simulink model "plant"  (R2015b)
settings: Solver=FixedStepAuto  StartTime=0.0  StopTime=10  FixedStep=0.001  RelTol=1e-3
values from neighbouring files (symbols this model uses):
  butterworthOrder = 1    [prerunScript.m]
  FP_c = x(1,1)    [checkPFvsL.m]    (also in passForceParams.m = 0.000395332869306)
  FP_k = x(1,2)    [checkPFvsL.m]    (also in passForceParams.m = 0.132380005179)
  FP_lr = x(1,3)    [checkPFvsL.m]    (also in passForceParams.m = -0.491551555037)
  lambda0 = [[0.00350486];[0.06666161];[0.14223155];[0.17875788];[0.09072633];[0.19503137];[0.07421535];[0.06014449];[0.07737726];[0.15431079];[0.05739210];[0.08251990];[0.05507007];[0.05698303];[0.06408346];[0.06303047];[0.05043992];[0.06209895];[0.05972867];[0.06428054];[0.05550584];[0.06070605];[0.04113306];[0.06599153];[0.06665474];[0.06653758];[0.07028198];[0.07750712];[0.04229977];[0.06486173];[0.064262 ...(+251 chars)    [prerunScript.m]
  ldotECoeffs = ldotCoeffs.ldotE    [prerunScript.m]
  ldotSCoeffs = ldotCoeffs.ldotS    [prerunScript.m]
  optimalLambda = [[0.027];[0.0713];[0.1157];[0.1321];[0.0858];[0.1726];      [0.0932];[0.0976];[0.1078];[0.1367];[0.0585];[0.081];[0.0622];[0.07];      [0.065];[0.0724];[0.0626];[0.0675];[0.0589];[0.0675];[0.054];[0.0628];      [0.0509];[0.0749];[0.0749];[0.0835];[0.0798];[0.0835];[0.0515];[0.0749];      [0.0736];[0.0552];[0.0755];[0.254];[0.2324];[0.2789];[0.1442];[0.1385];      [0.1385];[0.0638];[0.0282];[0.0492 ...(+78 chars)    [checkPFvsL.m]    (also in prerunScript.m)
  rhoECoeffs = zeros(50,degree+1)    [fit_moments.m]    (also in prerunScript.m = rhoCoeffs.rhoECoeffs; rhoCoeffs.mat = [1.24545301291e-20 0 -1.29464465569e-20 -1.29464465569e-20 -)
  rhoSCoeffs = zeros(50,degree+1)    [fit_moments.m]    (also in prerunScript.m = rhoCoeffs.rhoSCoeffs; rhoCoeffs.mat = [0 0 -4.82961585868e-21 1.75624779335e-24 0 0 1.43054523333e)
  uANC_p_a = 0    [setPCurla.m]    (also in setPRest.m; setPRestSLock.m; setPSweep.m)
  uANC_p_d = 1    [setPCurla.m]    (also in setPRest.m; setPRestSLock.m; setPSweep.m)
  uANC_p_p = 10    [setPCurla.m]    (also in setPRest.m; setPRestSLock.m; setPSweep.m)
  uANC_p_w = 20    [setPCurla.m]    (also in setPRest.m; setPRestSLock.m; setPSweep.m)
  uBRD_a = 25    [setPCurla.m]    (also in setPRest.m = 0; setPRestSLock.m = 0; setPSweep.m = 5; setPTPEC2.m = 0)
  uBRD_b = 0    [setPCurla.m]    (also in setPRest.m; setPRestSLock.m; setPSweep.m; setPTPEC2.m)
  uBRD_f = pi/10*3    (= 0.942477796077)    [setPCurla.m]    (also in setPRest.m; setPRestSLock.m; setPSweep.m; setPTPEC2.m)
  uBRD_p = 0    [setPCurla.m]    (also in setPRest.m; setPRestSLock.m; setPSweep.m; setPTPEC2.m)
  uTRIlong_a = 1140    [setPCurla.m]    (also in setPRest.m = 0; setPRestSLock.m = 0; setPSweep.m = 0; setPTPEC2.m = 0)
  uTRIlong_b = 0    [setPCurla.m]    (also in setPRest.m; setPRestSLock.m; setPSweep.m; setPTPEC2.m)
  uTRIlong_f = pi/10*3    (= 0.942477796077)    [setPCurla.m]    (also in setPRest.m; setPRestSLock.m; setPSweep.m; setPTPEC2.m)
  uTRIlong_p = pi    (= 3.14159265359)    [setPCurla.m]    (also in setPRest.m; setPRestSLock.m; setPSweep.m; setPTPEC2.m)
libraries: dsparch4 x50
settings Model: Creator=awni1  LastModifiedBy=hawni
settings DataIOCC: LimitDataPoints=off  SaveFormat=Array
settings HardwareCC: ProdBitPerPointer=32  ProdLargestAtomicFloat=None  ProdIntDivRoundTo=Undefined  ProdEndianess=Unspecified  ProdWordSize=32  ProdHWDeviceType=32-bit Generic
settings GRTTargetCC: GeneratePreprocessorConditionals=Disable all
settings ConfigComp: CovModelRefEnable=Off

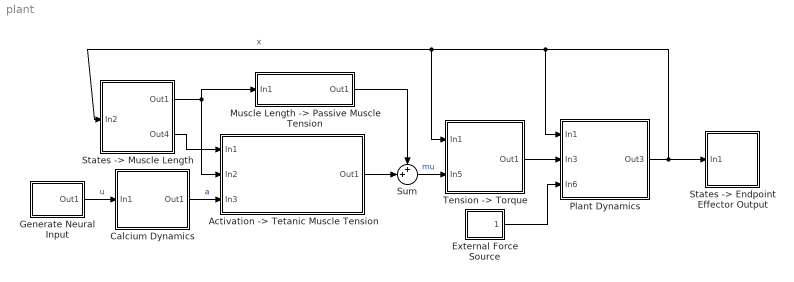
== system plant ==
  "Activation -> Tetanic Muscle Tension" : Subsystem
  Calcium Dynamics : Subsystem
  External Force Source : Subsystem
  Generate Neural Input : Subsystem
  "Muscle Length -> Passive Muscle Tension" : Subsystem
  Plant Dynamics : Subsystem
  "States -> Endpoint Effector Output" : Subsystem
  "States -> Muscle Length" : Subsystem
  Sum : Sum  Inputs=++|
  "Tension -> Torque" : Subsystem
  wires:
  Plant Dynamics/1(Out3) -> "States -> Muscle Length"/1(In2), "Tension -> Torque"/1(In1), Plant Dynamics/1(In1), "States -> Endpoint Effector Output"/1(In1)  "x"
  Calcium Dynamics/1(Out1) -> "Activation -> Tetanic Muscle Tension"/3(In3)  "a"
  "Activation -> Tetanic Muscle Tension"/1(Out1) -> Sum/2
  "States -> Muscle Length"/1(Out1) -> "Muscle Length -> Passive Muscle Tension"/1(In1), "Activation -> Tetanic Muscle Tension"/2(In2)
  "States -> Muscle Length"/2(Out4) -> "Activation -> Tetanic Muscle Tension"/1(In1)
  "Muscle Length -> Passive Muscle Tension"/1(Out1) -> Sum/1
  Sum/1 -> "Tension -> Torque"/2(In5)  "mu"
  "Tension -> Torque"/1(Out1) -> Plant Dynamics/2(In3)
  External Force Source/1(Out1) -> Plant Dynamics/3(In6)
  Generate Neural Input/1(Out1) -> Calcium Dynamics/1(In1)  "u"

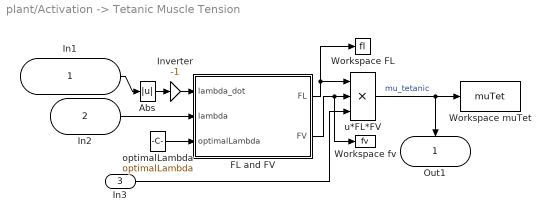
== system plant/Activation -> Tetanic Muscle Tension ==
  In1 : Inport
  In2 : Inport  Port=2
  In3 : Inport  Port=3
  Abs : Abs
  FL and FV : MATLAB Function  TreatAsAtomicUnit=on
  Inverter : Gain  Gain=-1
  Workspace FL : ToWorkspace  VariableName=fl  SampleTime=-1
  Workspace fv : ToWorkspace  VariableName=fv  SampleTime=-1
  Workspace muTet : ToWorkspace  VariableName=muTet  SampleTime=-1
  optimalLambda : Constant  Value=optimalLambda
  u*FL*FV : Product  Inputs=3
  Out1 : Outport
  wires:
  In2/1 -> FL and FV/2(lambda)
  In3/1 -> u*FL*FV/3
  In1/1 -> Abs/1
  FL and FV/1(FL) -> Workspace FL/1, u*FL*FV/1
  FL and FV/2(FV) -> Workspace fv/1, u*FL*FV/2
  optimalLambda/1 -> FL and FV/3(optimalLambda)
  Abs/1 -> Inverter/1
  Inverter/1 -> FL and FV/1(lambda_dot)
  u*FL*FV/1 -> Workspace muTet/1, Out1/1  "mu_tetanic"

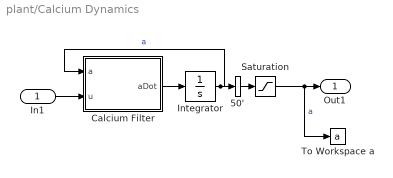
== system plant/Calcium Dynamics ==
  In1 : Inport
  50' : SignalSpecification  Dimensions=50
  Calcium Filter : MATLAB Function  TreatAsAtomicUnit=on
  Integrator : Integrator
  Saturation : Saturate  UpperLimit=inf  LowerLimit=0
  To Workspace a : ToWorkspace  VariableName=a  SampleTime=-1
  Out1 : Outport
  wires:
  In1/1 -> Calcium Filter/2(u)
  Saturation/1 -> To Workspace a/1, Out1/1  "a"
  50'/1 -> Saturation/1
  Calcium Filter/1(aDot) -> Integrator/1
  Integrator/1 -> Calcium Filter/1(a), 50'/1  "a"

== system plant/External Force Source ==
  Mux1 : Mux  Inputs=2
  Out1 : Outport
  wires:
  Mux1/1 -> Out1/1  "fE"

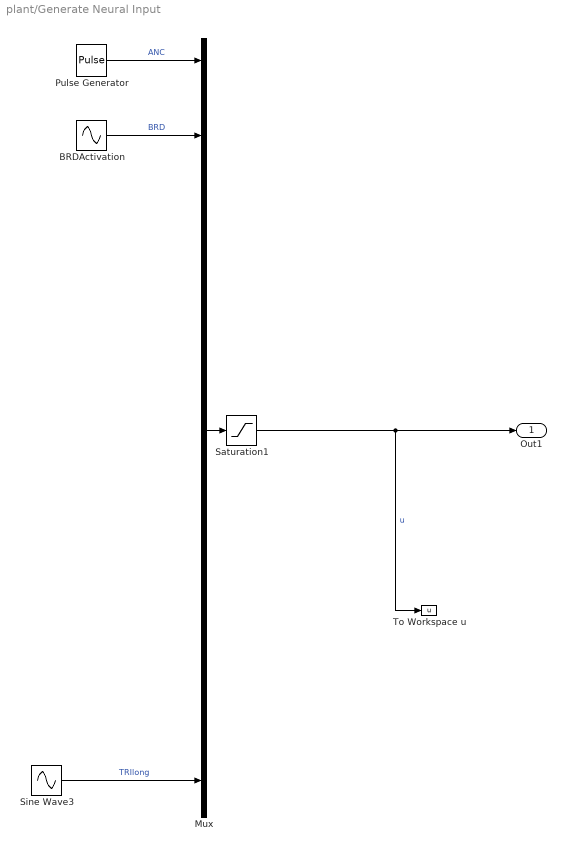
== system plant/Generate Neural Input ==
  BRDActivation : Sin  Amplitude=uBRD_a  Bias=uBRD_b  Frequency=uBRD_f  Phase=uBRD_p  SampleTime=0
  Mux : Mux  Inputs=50
  Pulse Generator : DiscretePulseGenerator  PulseType=Time based  Amplitude=uANC_p_a  Period=uANC_p_p  PulseWidth=uANC_p_w  PhaseDelay=uANC_p_d
  Saturation1 : Saturate  UpperLimit=1  LowerLimit=0
  Sine Wave3 : Sin  Amplitude=uTRIlong_a  Bias=uTRIlong_b  Frequency=uTRIlong_f  Phase=uTRIlong_p  SampleTime=0
  To Workspace u : ToWorkspace  VariableName=u  SampleTime=-1
  Out1 : Outport
  wires:
  ? -> Mux/41
  ? -> Mux/11
  ? -> Mux/23
  ? -> Mux/27
  ? -> Mux/3
  ? -> Mux/8
  ? -> Mux/29
  ? -> Mux/18
  ? -> Mux/19
  ? -> Mux/28
  ? -> Mux/26
  ? -> Mux/43
  ? -> Mux/33
  ? -> Mux/32
  ? -> Mux/17
  ? -> Mux/37
  ? -> Mux/42
  ? -> Mux/47
  ? -> Mux/48
  ? -> Mux/9
  ? -> Mux/16
  ? -> Mux/13
  ? -> Mux/4
  ? -> Mux/46
  ? -> Mux/22
  ? -> Mux/39
  ? -> Mux/7
  ? -> Mux/21
  ? -> Mux/24
  ? -> Mux/34
  ? -> Mux/44
  ? -> Mux/5
  ? -> Mux/15
  ? -> Mux/25
  ? -> Mux/35
  ? -> Mux/45
  ? -> Mux/38  "PEC2"
  Sine Wave3/1 -> Mux/49  "TRIlong"
  Pulse Generator/1 -> Mux/1  "ANC"
  Mux/1 -> Saturation1/1
  Saturation1/1 -> Out1/1, To Workspace u/1  "u"
  ? -> Mux/36
  ? -> Mux/2
  ? -> Mux/12
  ? -> Mux/31
  ? -> Mux/14
  BRDActivation/1 -> Mux/6  "BRD"

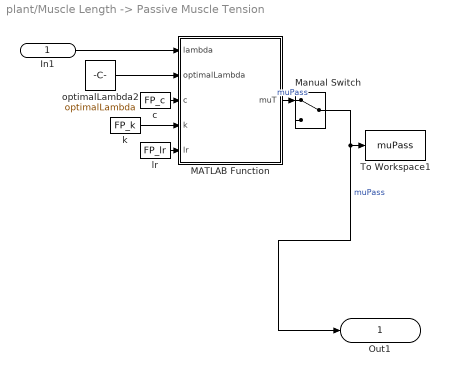
== system plant/Muscle Length -> Passive Muscle Tension ==
  In1 : Inport
  MATLAB Function : MATLAB Function  TreatAsAtomicUnit=on
  Manual Switch : ManualSwitch
  To Workspace1 : ToWorkspace  VariableName=muPass  SampleTime=-1
  c : Constant  Value=FP_c
  k : Constant  Value=FP_k
  lr : Constant  Value=FP_lr
  optimalLambda2 : Constant  Value=optimalLambda
  Out1 : Outport
  wires:
  In1/1 -> MATLAB Function/1(lambda)
  c/1 -> MATLAB Function/3(c)
  k/1 -> MATLAB Function/4(k)
  lr/1 -> MATLAB Function/5(lr)
  optimalLambda2/1 -> MATLAB Function/2(optimalLambda)
  MATLAB Function/1(muT) -> Manual Switch/1  "muPass"
  Manual Switch/1 -> Out1/1, To Workspace1/1  "muPass"

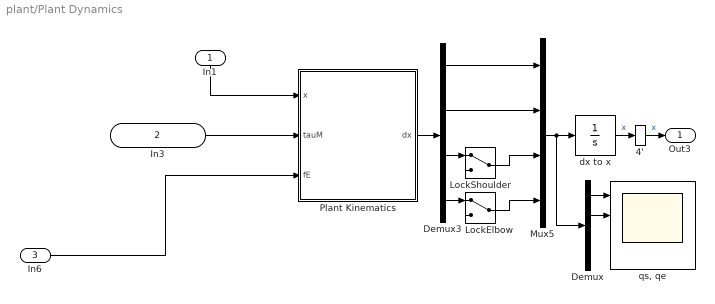
== system plant/Plant Dynamics ==
  In1 : Inport
  In3 : Inport  Port=2
  In6 : Inport  Port=3
  4' : SignalSpecification  Dimensions=4
  Demux : Demux
  Demux3 : Demux
  LockElbow : ManualSwitch
  LockShoulder : ManualSwitch
  Mux5 : Mux
  Plant Kinematics : MATLAB Function  TreatAsAtomicUnit=on
  dx to x : Integrator  InitialCondition=[90,0,0,0]
  "qs, qe" : Scope  NumInputPorts=4
  Out3 : Outport
  wires:
  In3/1 -> Plant Kinematics/2(tauM)
  In1/1 -> Plant Kinematics/1(x)
  In6/1 -> Plant Kinematics/3(fE)
  Plant Kinematics/1(dx) -> Demux3/1
  Demux3/4 -> LockElbow/1
  LockShoulder/1 -> Mux5/3
  Demux3/3 -> LockShoulder/1
  LockElbow/1 -> Mux5/4
  Demux3/1 -> Mux5/1
  Demux3/2 -> Mux5/2
  Demux/2 -> "qs, qe"/2
  Mux5/1 -> Demux/1, dx to x/1
  dx to x/1 -> 4'/1  "x"
  4'/1 -> Out3/1  "x"
  Demux/1 -> "qs, qe"/1

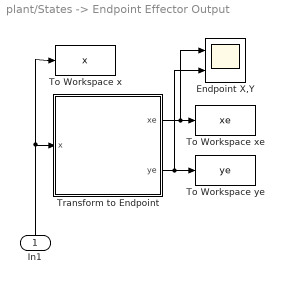
== system plant/States -> Endpoint Effector Output ==
  In1 : Inport
  Endpoint X,Y : Scope  NumInputPorts=2
  To Workspace x : ToWorkspace  VariableName=x  SampleTime=-1
  To Workspace xe : ToWorkspace  VariableName=xe  SampleTime=-1
  To Workspace ye : ToWorkspace  VariableName=ye  SampleTime=-1
  Transform to Endpoint : MATLAB Function  TreatAsAtomicUnit=on
  wires:
  In1/1 -> To Workspace x/1, Transform to Endpoint/1(x)
  Transform to Endpoint/1(xe) -> Endpoint X,Y/1, To Workspace xe/1
  Transform to Endpoint/2(ye) -> Endpoint X,Y/2, To Workspace ye/1

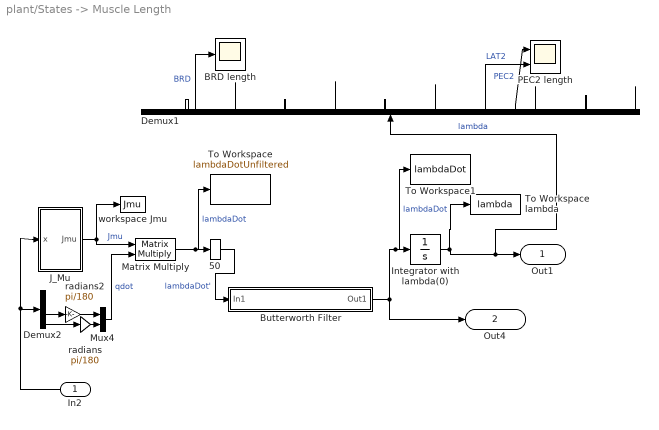
== system plant/States -> Muscle Length ==
  In2 : Inport
  50 : SignalSpecification  Dimensions=50
  BRD length : Scope
  Butterworth Filter : Subsystem
  Demux1 : Demux  Outputs=50
  Demux2 : Demux
  Integrator with lambda(0) : Integrator  InitialCondition=lambda0
  J_Mu : Subsystem
  Matrix Multiply : Product  Multiplication=Matrix(*)
  Mux4 : Mux  Inputs=2
  PEC2 length : Scope  NumInputPorts=2
  To Workspace : ToWorkspace  VariableName=lambdaDotUnfiltered  SampleTime=-1
  To Workspace lambda : ToWorkspace  VariableName=lambda  SampleTime=-1
  To Workspace1 : ToWorkspace  VariableName=lambdaDot  SampleTime=-1
  radians : Gain  Gain=pi/180
  radians2 : Gain  Gain=pi/180
  workspace Jmu : ToWorkspace  VariableName=Jmu  SampleTime=-1
  Out1 : Outport
  Out4 : Outport  Port=2
  wires:
  In2/1 -> Demux2/1, J_Mu/1(x)
  J_Mu/1(Jmu) -> workspace Jmu/1, Matrix Multiply/1  "Jmu"
  Mux4/1 -> Matrix Multiply/2  "qdot"
  Matrix Multiply/1 -> To Workspace/1, 50/1  "lambdaDot"
  Integrator with lambda(0)/1 -> To Workspace lambda/1, Demux1/1, Out1/1  "lambda"
  Demux2/3 -> radians2/1
  radians/1 -> Mux4/2
  radians2/1 -> Mux4/1
  Demux2/4 -> radians/1
  Demux1/6 -> BRD length/1  "BRD"
  Demux1/5 -> ?
  Demux1/10 -> ?
  Demux1/15 -> ?
  Demux1/20 -> ?
  Demux1/25 -> ?
  Demux1/30 -> ?
  Demux1/40 -> ?
  Demux1/45 -> ?
  Demux1/50 -> ?
  Demux1/38 -> PEC2 length/1  "PEC2"
  Demux1/35 -> PEC2 length/2  "LAT2"
  50/1 -> Butterworth Filter/1(In1)  "lambdaDot'"
  Butterworth Filter/1(Out1) -> Out4/1, To Workspace1/1, Integrator with lambda(0)/1  "lambdaDot"

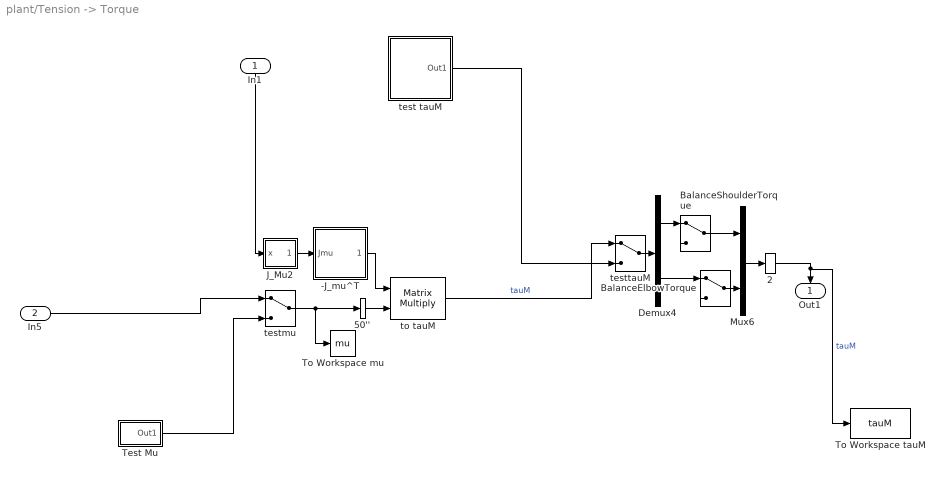
== system plant/Tension -> Torque ==
  In1 : Inport
  In5 : Inport  Port=2
  -J_mu^T : MATLAB Function  TreatAsAtomicUnit=on
  2 : SignalSpecification  Dimensions=2
  50'' : SignalSpecification  Dimensions=50
  BalanceElbowTorque : ManualSwitch
  BalanceShoulderTorque : ManualSwitch
  Demux4 : Demux  Outputs=2
  J_Mu2 : Subsystem
  Mux6 : Mux  Inputs=2
  Test Mu : Subsystem
  To Workspace mu : ToWorkspace  VariableName=mu  SampleTime=-1
  To Workspace tauM : ToWorkspace  VariableName=tauM  SampleTime=-1
  test tauM : Subsystem
  testmu : ManualSwitch
  testtauM : ManualSwitch
  to tauM : Product  Multiplication=Matrix(*)
  Out1 : Outport
  wires:
  In5/1 -> testmu/1
  In1/1 -> J_Mu2/1(x)
  2/1 -> To Workspace tauM/1, Out1/1  "tauM"
  testmu/1 -> 50''/1, To Workspace mu/1
  -J_mu^T/1(JmuT) -> to tauM/1
  J_Mu2/1(Jmu) -> -J_mu^T/1(Jmu)
  to tauM/1 -> testtauM/1  "tauM"
  50''/1 -> to tauM/2
  Mux6/1 -> 2/1
  testtauM/1 -> Demux4/1
  BalanceShoulderTorque/1 -> Mux6/1
  BalanceElbowTorque/1 -> Mux6/2
  Demux4/1 -> BalanceShoulderTorque/1
  Demux4/2 -> BalanceElbowTorque/1
  Test Mu/1(Out1) -> testmu/2
  test tauM/1(Out1) -> testtauM/2

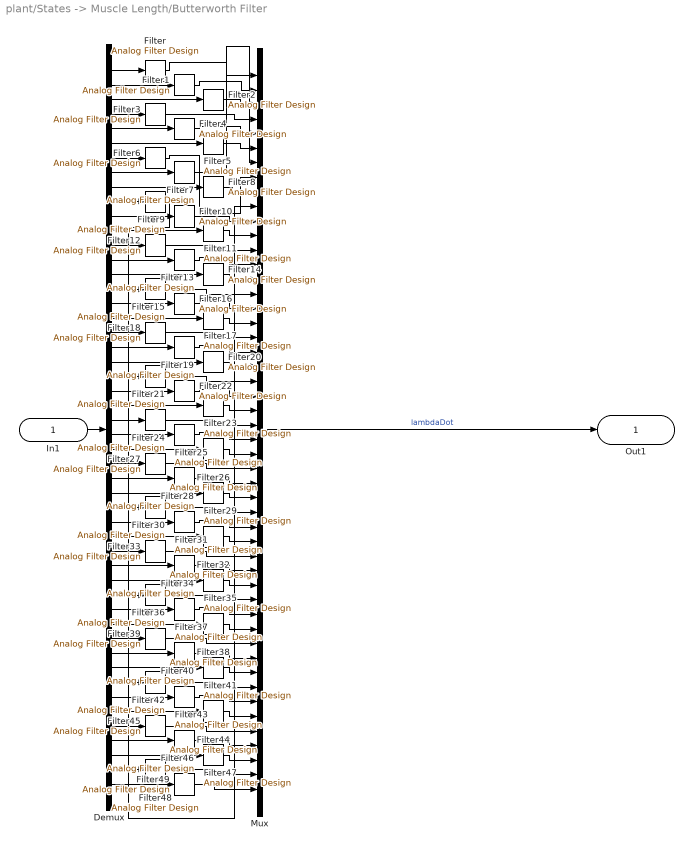
== system plant/States -> Muscle Length/Butterworth Filter ==
  In1 : Inport
  Demux : Demux  Outputs=50
  Filter{,1..49} (50 alike) : dsparch4/Analog Filter Design  method=Butterworth  filttype=Lowpass  N=butterworthOrder  Wlo=butterworthCutoffFreq  Whi=80  Rp=2  Rs=40
  Mux : Mux  Inputs=50
  Out1 : Outport
  wires:
  In1/1 -> Demux/1
  Demux/1 -> Filter/1
  Demux/2 -> Filter1/1
  Demux/3 -> Filter2/1
  Demux/4 -> Filter3/1
  Demux/5 -> Filter4/1
  Demux/6 -> Filter5/1
  Demux/9 -> Filter8/1
  Demux/8 -> Filter7/1
  Demux/7 -> Filter6/1
  Demux/10 -> Filter9/1
  Demux/11 -> Filter10/1
  Demux/12 -> Filter11/1
  Demux/13 -> Filter12/1
  Demux/14 -> Filter13/1
  Demux/15 -> Filter14/1
  Demux/16 -> Filter15/1
  Demux/17 -> Filter16/1
  Demux/18 -> Filter17/1
  Demux/19 -> Filter18/1
  Demux/20 -> Filter19/1
  Demux/21 -> Filter20/1
  Demux/22 -> Filter21/1
  Demux/23 -> Filter22/1
  Demux/24 -> Filter23/1
  Demux/26 -> Filter25/1
  Demux/25 -> Filter24/1
  Demux/27 -> Filter26/1
  Demux/28 -> Filter27/1
  Demux/29 -> Filter28/1
  Demux/30 -> Filter29/1
  Demux/31 -> Filter30/1
  Demux/32 -> Filter31/1
  Demux/33 -> Filter32/1
  Demux/34 -> Filter33/1
  Demux/35 -> Filter34/1
  Demux/36 -> Filter35/1
  Demux/37 -> Filter36/1
  Demux/38 -> Filter37/1
  Demux/39 -> Filter38/1
  Demux/40 -> Filter39/1
  Demux/41 -> Filter40/1
  Demux/42 -> Filter41/1
  Demux/43 -> Filter42/1
  Demux/44 -> Filter43/1
  Demux/45 -> Filter44/1
  Demux/47 -> Filter46/1
  Demux/46 -> Filter45/1
  Demux/48 -> Filter47/1
  Demux/49 -> Filter48/1
  Demux/50 -> Filter49/1
  Mux/1 -> Out1/1  "lambdaDot"
  Filter/1 -> Mux/1
  Filter1/1 -> Mux/2
  Filter2/1 -> Mux/3
  Filter3/1 -> Mux/4
  Filter4/1 -> Mux/5
  Filter5/1 -> Mux/6
  Filter6/1 -> Mux/7
  Filter7/1 -> Mux/8
  Filter8/1 -> Mux/9
  Filter9/1 -> Mux/10
  Filter10/1 -> Mux/11
  Filter11/1 -> Mux/12
  Filter12/1 -> Mux/13
  Filter13/1 -> Mux/14
  Filter14/1 -> Mux/15
  Filter15/1 -> Mux/16
  Filter16/1 -> Mux/17
  Filter17/1 -> Mux/18
  Filter18/1 -> Mux/19
  Filter19/1 -> Mux/20
  Filter20/1 -> Mux/21
  Filter21/1 -> Mux/22
  Filter22/1 -> Mux/23
  Filter23/1 -> Mux/24
  Filter24/1 -> Mux/25
  Filter25/1 -> Mux/26
  Filter26/1 -> Mux/27
  Filter27/1 -> Mux/28
  Filter28/1 -> Mux/29
  Filter29/1 -> Mux/30
  Filter30/1 -> Mux/31
  Filter31/1 -> Mux/32
  Filter32/1 -> Mux/33
  Filter33/1 -> Mux/34
  Filter34/1 -> Mux/35
  Filter35/1 -> Mux/36
  Filter36/1 -> Mux/37
  Filter37/1 -> Mux/38
  Filter38/1 -> Mux/39
  Filter39/1 -> Mux/40
  Filter40/1 -> Mux/41
  Filter41/1 -> Mux/42
  Filter42/1 -> Mux/43
  Filter43/1 -> Mux/44
  Filter44/1 -> Mux/45
  Filter45/1 -> Mux/46
  Filter46/1 -> Mux/47
  Filter47/1 -> Mux/48
  Filter48/1 -> Mux/49
  Filter49/1 -> Mux/50

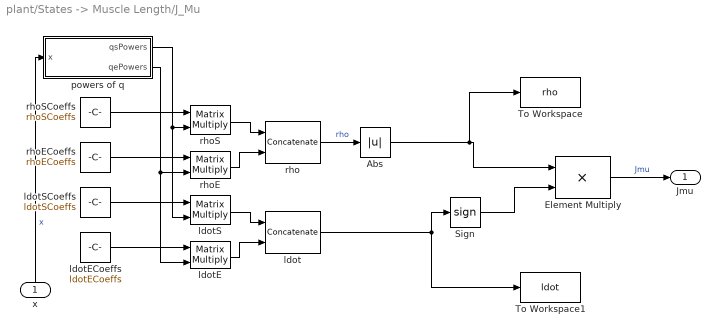
== system plant/States -> Muscle Length/J_Mu ==
  x : Inport  PortDimensions=4
  Abs : Abs
  Element Multiply : Product
  Sign : Signum
  To Workspace : ToWorkspace  VariableName=rho  SampleTime=-1
  To Workspace1 : ToWorkspace  VariableName=ldot  SampleTime=-1
  ldot : Concatenate  Mode=Multidimensional array  ConcatenateDimension=2
  ldotE : Product  Multiplication=Matrix(*)
  ldotECoeffs : Constant  Value=ldotECoeffs
  ldotS : Product  Multiplication=Matrix(*)
  ldotSCoeffs : Constant  Value=ldotSCoeffs
  powers of q : MATLAB Function  TreatAsAtomicUnit=on
  rho : Concatenate  Mode=Multidimensional array  ConcatenateDimension=2
  rhoE : Product  Multiplication=Matrix(*)
  rhoECoeffs : Constant  Value=rhoECoeffs
  rhoS : Product  Multiplication=Matrix(*)
  rhoSCoeffs : Constant  Value=rhoSCoeffs
  Jmu : Outport
  wires:
  powers of q/1(qsPowers) -> ldotS/2, rhoS/2
  rhoECoeffs/1 -> rhoE/1
  powers of q/2(qePowers) -> ldotE/2, rhoE/2
  x/1 -> powers of q/1(x)  "x"
  rhoS/1 -> rho/1
  rhoSCoeffs/1 -> rhoS/1
  rhoE/1 -> rho/2
  ldotS/1 -> ldot/1
  ldotE/1 -> ldot/2
  ldotSCoeffs/1 -> ldotS/1
  ldotECoeffs/1 -> ldotE/1
  Element Multiply/1 -> Jmu/1  "Jmu"
  ldot/1 -> Sign/1, To Workspace1/1
  rho/1 -> Abs/1  "rho"
  Abs/1 -> To Workspace/1, Element Multiply/1
  Sign/1 -> Element Multiply/2

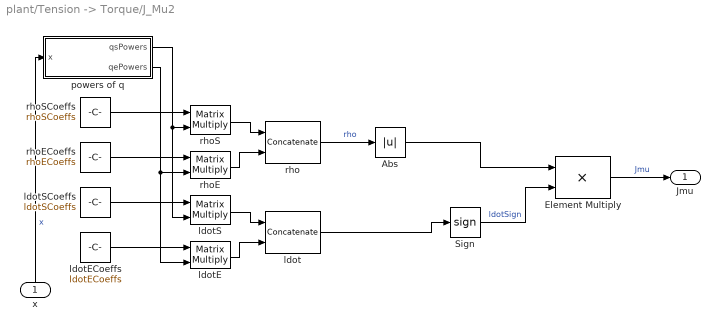
== system plant/Tension -> Torque/J_Mu2 ==
  x : Inport  PortDimensions=4
  Abs : Abs
  Element Multiply : Product
  Sign : Signum
  ldot : Concatenate  Mode=Multidimensional array  ConcatenateDimension=2
  ldotE : Product  Multiplication=Matrix(*)
  ldotECoeffs : Constant  Value=ldotECoeffs
  ldotS : Product  Multiplication=Matrix(*)
  ldotSCoeffs : Constant  Value=ldotSCoeffs
  powers of q : MATLAB Function  TreatAsAtomicUnit=on
  rho : Concatenate  Mode=Multidimensional array  ConcatenateDimension=2
  rhoE : Product  Multiplication=Matrix(*)
  rhoECoeffs : Constant  Value=rhoECoeffs
  rhoS : Product  Multiplication=Matrix(*)
  rhoSCoeffs : Constant  Value=rhoSCoeffs
  Jmu : Outport
  wires:
  powers of q/1(qsPowers) -> ldotS/2, rhoS/2
  rhoECoeffs/1 -> rhoE/1
  powers of q/2(qePowers) -> ldotE/2, rhoE/2
  x/1 -> powers of q/1(x)  "x"
  rhoS/1 -> rho/1
  rhoSCoeffs/1 -> rhoS/1
  rhoE/1 -> rho/2
  ldotS/1 -> ldot/1
  ldotE/1 -> ldot/2
  ldotSCoeffs/1 -> ldotS/1
  ldotECoeffs/1 -> ldotE/1
  Sign/1 -> Element Multiply/2  "ldotSign"
  Element Multiply/1 -> Jmu/1  "Jmu"
  ldot/1 -> Sign/1
  rho/1 -> Abs/1  "rho"
  Abs/1 -> Element Multiply/1

== system plant/Tension -> Torque/Test Mu ==
  Manual Switch : ManualSwitch  CurrentSetting=0
  Mux3 : Mux  Inputs=50
  Sine Wave1 : Sin  Frequency=2*pi/10  SampleTime=0
  Step1 : Step  Time=0  After=0  SampleTime=0
  Sum1 : Sum  Inputs=++|
  Out1 : Outport
  wires:
  ? -> Mux3/42
  Mux3/1 -> Out1/1  "testMu"
  ? -> Mux3/49
  ? -> Mux3/7
  ? -> Mux3/41
  ? -> Mux3/30
  ? -> Mux3/29
  ? -> Mux3/15
  ? -> Mux3/22
  ? -> Mux3/44
  ? -> Mux3/4
  ? -> Mux3/16
  ? -> Mux3/23
  ? -> Mux3/43
  ? -> Mux3/20
  ? -> Mux3/2
  ? -> Mux3/5
  ? -> Mux3/21
  ? -> Mux3/1
  ? -> Mux3/33
  ? -> Mux3/34
  ? -> Mux3/19
  ? -> Mux3/32
  ? -> Mux3/31
  ? -> Mux3/14
  ? -> Mux3/8
  ? -> Mux3/11
  ? -> Mux3/18
  ? -> Mux3/17
  ? -> Mux3/40
  ? -> Mux3/12
  ? -> Mux3/28
  ? -> Mux3/13
  ? -> Mux3/50
  ? -> Mux3/24
  ? -> Mux3/9
  ? -> Mux3/35
  ? -> Mux3/47
  ? -> Mux3/10
  ? -> Mux3/25
  ? -> Mux3/39
  ? -> Mux3/26
  ? -> Mux3/37
  ? -> Mux3/38
  ? -> Mux3/27
  ? -> Mux3/36
  ? -> Mux3/45
  ? -> Mux3/48
  ? -> Mux3/46
  ? -> Mux3/3
  Step1/1 -> Sum1/1
  Sine Wave1/1 -> Sum1/2
  Manual Switch/1 -> Mux3/6  "BRD"
  Sum1/1 -> Manual Switch/1

== system plant/Tension -> Torque/test tauM ==
  Mux2 : Mux  Inputs=2
  tauS : Sin  Amplitude=0.02  Frequency=2*pi/10  SampleTime=0
  Out1 : Outport
  wires:
  Mux2/1 -> Out1/1  "test_tauM"
  tauS/1 -> Mux2/2

== matlab function plant/States -> Endpoint Effector Output/Transform to Endpoint ==
  data: x input; xe output; ye output
function [xe,ye]= toEndEffectorXY(x)
% init
    Ls=0.31;
    Le=0.34;
% translate
xe = cos((x(1)*pi/180))*Ls+Le*cos((x(1)*pi/180)+(x(2)*pi/180));
ye = sin((x(1)*pi/180))*Ls+Le*sin((x(1)*pi/180)+(x(2)*pi/180));

== matlab function plant/Plant Dynamics/Plant Kinematics ==
  data: x input; dx output; tauM input; fE input
function dx = armKinematics(x, tauM, fE)
    % define constants
    is=0.0141;
    ie=0.0188;
    lms=0.165;
    lme=0.19;
    Ls=0.31;
    Le=0.34;
    ms=1.93;
    me=1.52;

    % define dx as a vector 
    dx=zeros(4,1);
    
    dx(1) = x(3);
    dx(2) = x(4);
    dx(3) = -((fE(1)*ie - fE(2)*ie + fE(1)*is + fE(1)*lme^2*me - fE(2)*lme^2 * ...
        me + fE(1)*Ls^2*me + fE(1)*lms^2*ms + ie*tauM(1) + is*tauM(1) + ... 
        lme^2*me*tauM(1) + Ls^2*me*tauM(1) + lms^2*ms*tauM(1) - ie* ...
        tauM(2) - lme^2*me*tauM(2) + fE(1)*lme*Ls*me*cos((x(2)*pi/180)) - fE(2) ...
        *lme*Ls*me*cos((x(2)*pi/180)) + lme*Ls*me*tauM(1)*cos((x(2)*pi/180)) - lme*Ls*me* ...
        tauM(2)*cos((x(2)*pi/180)) + ie*lme*Ls*me*((x(4)*pi/180))^2*sin((x(2)*pi/180)) + is*lme*Ls* ...
        me*((x(4)*pi/180))^2*sin((x(2)*pi/180)) + lme^3*Ls*me^2*((x(4)*pi/180))^2*sin((x(2)*pi/180)) + lme* ...
        Ls^3*me^2*((x(4)*pi/180))^2*sin((x(2)*pi/180)) + lme*lms^2*Ls*me*ms*((x(4)*pi/180))^2*sin((x(2)*pi/180)) ...
        + 2*ie*lme*Ls*me*((x(4)*pi/180))*((x(3)*pi/180))*sin((x(2)*pi/180)) + 2*is*lme*Ls*me*((x(4)*pi/180))* ...
        ((x(3)*pi/180))*sin((x(2)*pi/180)) + 2*lme^3*Ls*me^2*((x(4)*pi/180))*((x(3)*pi/180))*sin((x(2)*pi/180)) + ...
        2*lme*Ls^3*me^2*((x(4)*pi/180))*((x(3)*pi/180))*sin((x(2)*pi/180)) + 2*lme*lms^2*Ls*me*ms* ...
        ((x(4)*pi/180))*((x(3)*pi/180))*sin((x(2)*pi/180)) + ie*lme*Ls*me*((x(3)*pi/180))^2*sin((x(2)*pi/180)) + lme^3* ...
        Ls*me^2*((x(3)*pi/180))^2*sin((x(2)*pi/180)) + lme^2*Ls^2*me^2*((x(4)*pi/180))^2*cos((x(2)*pi/180))*sin((x(2)*pi/180)) ...
        + 2*lme^2*Ls^2*me^2*((x(4)*pi/180))*((x(3)*pi/180))*cos((x(2)*pi/180))*sin((x(2)*pi/180)) + ...
        lme^2*Ls^2*me^2*((x(3)*pi/180))^2*cos((x(2)*pi/180))*sin((x(2)*pi/180)))/(-ie*is - is*lme^2*me ...
        - ie*Ls^2*me - lme^2*Ls^2*me^2 - ie*lms^2*ms - lme^2*lms^2*me*ms + ...
        ie*lme*Ls*me*cos((x(2)*pi/180)) + lme^3*Ls*me^2*cos((x(2)*pi/180)) + lme^2*Ls^2*me^2 ...
        *cos((x(2)*pi/180))^2));
    dx(4) = -((-(-ie - lme^2*me - lme*Ls*me*cos((x(2)*pi/180)))*(fE(1) + tauM(1) + ...
        lme*Ls*me*((x(4)*pi/180))^2*sin((x(2)*pi/180)) + 2*lme*Ls*me*((x(4)*pi/180))*((x(3)*pi/180))*sin((x(2)*pi/180))) ...
        + (-ie - lme^2*me)*(fE(2) + tauM(2) - lme*Ls*me*((x(3)*pi/180))^2*sin((x(2)*pi/180)))) ...
        /(-(-ie - lme^2*me - lme*Ls*me*cos((x(2)*pi/180)))^2 + (-ie - lme^2*me) * ...
        (-ie - is - lme^2*me - Ls^2*me - lms^2*ms - lme*Ls*me*cos((x(2)*pi/180)))));

% With only x(1) and x(2) scaled
% function dx = armKinematics(x, tauM, fE)
%     % define constants
%     is=0.0141;
%     ie=0.0188;
%     lms=0.165;
%     lme=0.19;
%     Ls=0.31;
%     Le=0.34;
%     ms=1.93;
%     me=1.52;
% 
%     % define dx as a vector 
%     dx=zeros(4,1);
%     
%     dx(1) = x(3);
%     dx(2) = x(4);
%     dx(3) = -((fE(1)*ie - fE(2)*ie + fE(1)*is + fE(1)*lme^2*me - fE(2)*lme^2 * ...
%         me + fE(1)*Ls^2*me + fE(1)*lms^2*ms + ie*tauM(1) + is*tauM(1) + ... 
%         lme^2*me*tauM(1) + Ls^2*me*tauM(1) + lms^2*ms*tauM(1) - ie* ...
%         tauM(2) - lme^2*me*tauM(2) + fE(1)*lme*Ls*me*cos((x(2)*pi/180)) - fE(2) ...
%         *lme*Ls*me*cos((x(2)*pi/180)) + lme*Ls*me*tauM(1)*cos((x(2)*pi/180)) - lme*Ls*me* ...
%         tauM(2)*cos((x(2)*pi/180)) + ie*lme*Ls*me*(x(4))^2*sin((x(2)*pi/180)) + is*lme*Ls* ...
%         me*(x(4))^2*sin((x(2)*pi/180)) + lme^3*Ls*me^2*(x(4))^2*sin((x(2)*pi/180)) + lme* ...
%         Ls^3*me^2*(x(4))^2*sin((x(2)*pi/180)) + lme*lms^2*Ls*me*ms*(x(4))^2*sin((x(2)*pi/180)) ...
%         + 2*ie*lme*Ls*me*(x(4))*(x(3))*sin((x(2)*pi/180)) + 2*is*lme*Ls*me*(x(4))* ...
%         (x(3))*sin((x(2)*pi/180)) + 2*lme^3*Ls*me^2*(x(4))*(x(3))*sin((x(2)*pi/180)) + ...
%         2*lme*Ls^3*me^2*(x(4))*(x(3))*sin((x(2)*pi/180)) + 2*lme*lms^2*Ls*me*ms* ...
%         (x(4))*(x(3))*sin((x(2)*pi/180)) + ie*lme*Ls*me*(x(3))^2*sin((x(2)*pi/180)) + lme^3* ...
%         Ls*me^2*(x(3))^2*sin((x(2)*pi/180)) + lme^2*Ls^2*me^2*(x(4))^2*cos((x(2)*pi/180))*sin((x(2)*pi/180)) ...
%         + 2*lme^2*Ls^2*me^2*(x(4))*(x(3))*cos((x(2)*pi/180))*sin((x(2)*pi/180)) + ...
%         lme^2*Ls^2*me^2*(x(3))^2*cos((x(2)*pi/180))*sin((x(2)*pi/180)))/(-ie*is - is*lme^2*me ...
%         - ie*Ls^2*me - lme^2*Ls^2*me^2 - ie*lms^2*ms - lme^2*lms^2*me*ms + ...
%         ie*lme*Ls*me*cos((x(2)*pi/180)) + lme^3*Ls*me^2*cos((x(2)*pi/180)) + lme^2*Ls^2*me^2 ...
%         *cos((x(2)*pi/180))^2));
%     dx(4) = -((-(-ie - lme^2*me - lme*Ls*me*cos((x(2)*pi/180)))*(fE(1) + tauM(1) + ...
%         lme*Ls*me*(x(4))^2*sin((x(2)*pi/180)) + 2*lme*Ls*me*(x(4))*(x(3))*sin((x(2)*pi/180))) ...
%         + (-ie - lme^2*me)*(fE(2) + tauM(2) - lme*Ls*me*(x(3))^2*sin((x(2)*pi/180)))) ...
%         /(-(-ie - lme^2*me - lme*Ls*me*cos((x(2)*pi/180)))^2 + (-ie - lme^2*me) * ...
%         (-ie - is - lme^2*me - Ls^2*me - lms^2*ms - lme*Ls*me*cos((x(2)*pi/180)))));
%

== matlab function plant/Tension -> Torque/-J_mu^T ==
  data: Jmu input; JmuT output
function JmuT = transpose(Jmu)
JmuT = -1*Jmu.';

== matlab function plant/Activation -> Tetanic Muscle Tension/FL and FV ==
  data: lambda_dot input; lambda input; FL output; FV output; optimalLambda input
function [FL,FV] = toMuscleEffects(lambda_dot,lambda,optimalLambda)
nMuscles = 50;

% FL
beta = 1.93;
omega = 1.03;
rho = 1.87;

% FV
cv0 = 1.38;
cv1 = 2.09;
vMax = -5.72;
bv = 0.62;
av0 = -3.12;
av1 = 4.21;
av2 = -2.67;

% Construction
FL = zeros(nMuscles,1);
FV = zeros(nMuscles,1);
for i = 1:nMuscles
    FL(i,1) = exp(-abs(((lambda(i,1)/optimalLambda(i,1))^beta-1)/omega)^rho);
    if(lambda_dot(i) <= 0)
        FV(i,1) = (vMax - (lambda_dot(i)/optimalLambda(i,1)))/(vMax + (cv0 + ...
            cv1*(lambda(i)/optimalLambda(i,1)))*lambda_dot(i)/optimalLambda(i,1));
    else
        FV(i,1) = (bv - (av0+av1*lambda(i)/optimalLambda(i,1) +  ...
            av2*(lambda(i)/optimalLambda(i,1))^2)*lambda_dot(i)/optimalLambda(i,1))/ ...
            (bv + lambda_dot(i)/optimalLambda(i,1));
    end
end

%% Debugging
% nMuscles = 50;
% optimalLambda = [[0.027];[0.0713];[0.1157];[0.1321];[0.0858];[0.1726]; ...
%     [0.0932];[0.0976];[0.1078];[0.1367];[0.0585];[0.081];[0.0622];[0.07]; ...
%     [0.065];[0.0724];[0.0626];[0.0675];[0.0589];[0.0675];[0.054];[0.0628]; ...
%     [0.0509];[0.0749];[0.0749];[0.0835];[0.0798];[0.0835];[0.0515];[0.0749]; ...
%     [0.0736];[0.0552];[0.0755];[0.254];[0.2324];[0.2789];[0.1442];[0.1385]; ...
%     [0.1385];[0.0638];[0.0282];[0.0492];[0.0873];[0.033];[0.0682];[0.1624]; ...
%     [0.0741];[0.1138];[0.134];[0.1138]];
% 
% % FL
% beta = 1.93;
% omega = 1.03;
% rho = 1.87;
% 
% % FV
% cv0 = 1.38;
% cv1 = 2.09;
% vMax = -5.72;
% bv = 0.62;
% av0 = -3.12;
% av1 = 4.21;
% av2 = -2.67;
% 
% % Construction
% nstop = 741
% FL = ones(nMuscles,10001);
% FV = ones(nMuscles,10001);
% for i = 1:nMuscles 
% for j = 1:10001
%     FL(i,j) = exp(-abs(((lambda(j,i)/optimalLambda(i,1))^beta-1)/omega)^rho);
%     if(lambdaDot(j,i) <= 0)
%         FV(i,j) = (vMax - (lambdaDot(j,i)/optimalLambda(i,1)))/(vMax + (cv0 + ...
%             cv1*(lambda(j,i)/optimalLambda(i,1)))*lambdaDot(j,i)/optimalLambda(i,1));
%     else
%         FV(i,j) = (bv - (av0+av1*lambda(j,i)/optimalLambda(i,1) +  ...
%             av2*(lambda(j,i)/optimalLambda(i,1))^2)*lambdaDot(j,i)/optimalLambda(i,1))/ ...
%             (bv + lambdaDot(j,i)/optimalLambda(i,1));
%     end
% end
% end

== matlab function plant/Tension -> Torque/J_Mu2/powers of q ==
  data: x input; qsPowers output; qePowers output
function [qsPowers,qePowers] = pow(x)
%#codegen
degree = 10; %degree of fit of moment
qsPowers = zeros(degree+1,1);
qePowers = zeros(degree+1,1);
for i = (degree+1):-1:1
        qsPowers(degree+2-i,1) = (x(1))^(i-1);
        qePowers(degree+2-i,1) = (x(2))^(i-1);
end

== matlab function plant/States -> Muscle Length/J_Mu/powers of q ==
  data: x input; qsPowers output; qePowers output
function [qsPowers,qePowers] = pow(x)
%#codegen
degree = 10; %degree of fit of moment
qsPowers = zeros(degree+1,1);
qePowers = zeros(degree+1,1);
for i = (degree+1):-1:1
        qsPowers(degree+2-i,1) = (x(1))^(i-1);
        qePowers(degree+2-i,1) = (x(2))^(i-1);
end

== matlab function plant/Calcium Dynamics/Calcium Filter ==
  data: a input; u input; aDot output
function aDot = uToA(a,u)
tAct = 0.050;
tDeact = 0.066;
aDot = zeros(size(u,1),1);
for n = 1:size(u,1)
    t = 1;
    if u(n) > a(n)
        t = tDeact + u(n) * (tAct - tDeact);
    else
        t = tDeact;
    end
    aDot(n) = (u(n) - a(n))/t;
end

== matlab function plant/Muscle Length -> Passive Muscle Tension/MATLAB Function ==
  data: lambda input; muT output; optimalLambda input; c input; k input; lr input
function muT = tendonTension(lambda,optimalLambda,c,k,lr)
ls = lambda./optimalLambda;
muT = 0.0001*c*k*(exp((ls - lr)/k) + 1);
